simulink model "MAS_pc_up"  (R2022b)
settings: Solver=VariableStepAuto  StartTime=0.0  StopTime=300  RelTol=1e-3
values from neighbouring files (symbols this model uses):
  a1 = int8(3)    [init.m]
  A1 = [1.7,-1.3 ... (first row only)    [init.m]
  A2 = [1.8,-1.4 ... (first row only)    [init.m]
  a2 = int8(2)    [init.m]
  A3 = [1.4,-1.1 ... (first row only)    [init.m]
  a3 = int8(3)    [init.m]
  B1 = [1.0 ... (first row only)    [init.m]
  B2 = [1.7 ... (first row only)    [init.m]
  B3 = [0.8 ... (first row only)    [init.m]
  C1 = [1.0,0.3]    [init.m]
  C2 = [0.7,0.2]    [init.m]
  C3 = [1.1,0.4]    [init.m]
  F1 = [-0.4483 ... (first row only)    [init.m]
  F2 = [-0.6803 ... (first row only)    [init.m]
  F3 = [-0.3908 ... (first row only)    [init.m]
  G1 = -0.16    [init.m]
  G2 = -0.18    [init.m]
  G3 = -0.14    [init.m]
  H1 = -0.12    [init.m]
  H2 = -0.10    (= -0.1)    [init.m]
  H3 = -0.14    [init.m]
  M = [1,0,1 ... (first row only)    [init.m]
  s1 = int8(2)    [init.m]
  s2 = int8(3)    [init.m]
  s3 = int8(1)    [init.m]
  samp_t = 0.2    [init.m]
(part 1 of 2)
settings Model: Creator=Longct0  LastModifiedBy=Longct0

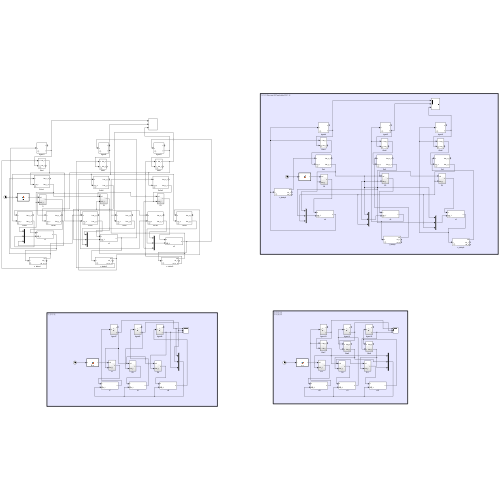
[thumbnail: Simulink's stored preview of the top-level diagram]
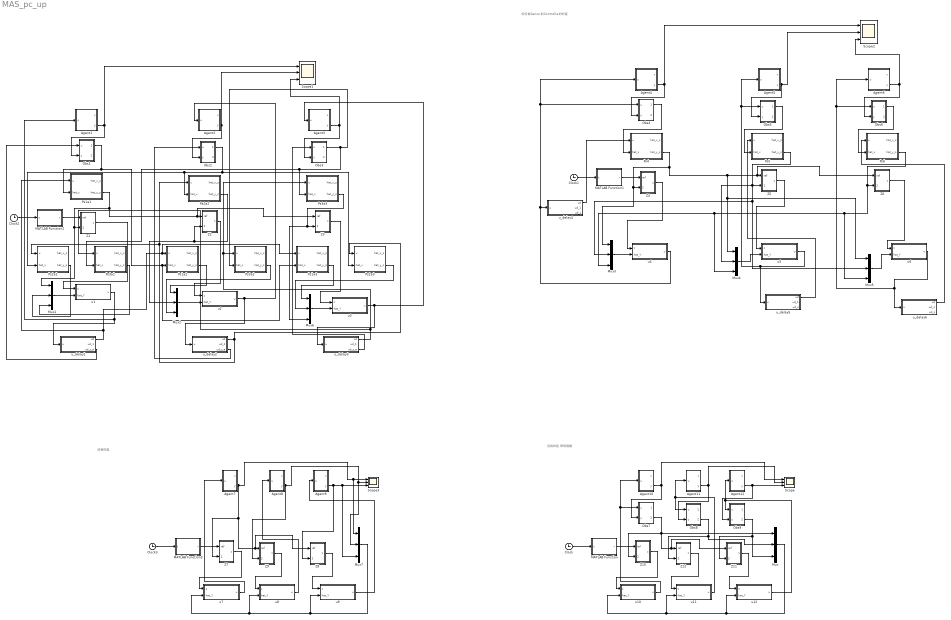
== system MAS_pc_up ==
  note: 仅仅有Sensor到Controller的时延
  note: 没有时延
      | 带观测器
  note: 没有时延
  Agent1 : Subsystem  mask{s=s1, a=a1}
      mask prompts: s "s-c"; a "c-a"
      mask DialogControl ParameterGroupVar Prompt: 参数
  Agent10 : Subsystem
  Agent11 : Subsystem
  Agent12 : Subsystem
  Agent2 : Subsystem  mask{s=s2, a=a2}
      mask prompts: s "s-c"; a "c-a"
      mask DialogControl ParameterGroupVar Prompt: 参数
  Agent3 : Subsystem  mask{s=s3, a=a3}
      mask prompts: s "s-c"; a "c-a"
      mask DialogControl ParameterGroupVar Prompt: 参数
  Agent4 : Subsystem  mask{s=s1, a=0}
      mask prompts: s "s-c"; a "c-a"
      mask DialogControl ParameterGroupVar Prompt: 参数
  Agent5 : Subsystem  mask{s=s2, a=0}
      mask prompts: s "s-c"; a "c-a"
      mask DialogControl ParameterGroupVar Prompt: 参数
  Agent6 : Subsystem  mask{s=s3, a=0}
      mask prompts: s "s-c"; a "c-a"
      mask DialogControl ParameterGroupVar Prompt: 参数
  Agent7 : Subsystem
  Agent8 : Subsystem
  Agent9 : Subsystem
  Clock{,1..3} (4 alike) : Clock
  MATLAB Function : MATLAB Function  TreatAsAtomicUnit=on
  MATLAB Function1 : MATLAB Function  TreatAsAtomicUnit=on
  MATLAB Function2 : MATLAB Function  TreatAsAtomicUnit=on
  MATLAB Function3 : MATLAB Function  TreatAsAtomicUnit=on
  Mux{,1..7} (8 alike) : Mux  Inputs=3
  Obs1 : Subsystem  mask{s=s1, a=a1}
      mask prompts: s "s-c"; a "c-a"
      mask DialogControl ParameterGroupVar Prompt: 参数
  Obs2 : Subsystem  mask{s=s2, a=a2}
      mask prompts: s "s-c"; a "c-a"
      mask DialogControl ParameterGroupVar Prompt: 参数
  Obs3 : Subsystem  mask{s=s3, a=a3}
      mask prompts: s "s-c"; a "c-a"
      mask DialogControl ParameterGroupVar Prompt: 参数
  Obs4 : Subsystem  mask{s=s1, a=a1}
      mask prompts: s "s-c"; a "c-a"
      mask DialogControl ParameterGroupVar Prompt: 参数
  Obs5 : Subsystem  mask{s=s2, a=a2}
      mask prompts: s "s-c"; a "c-a"
      mask DialogControl ParameterGroupVar Prompt: 参数
  Obs6 : Subsystem  mask{s=s3, a=a3}
      mask prompts: s "s-c"; a "c-a"
      mask DialogControl ParameterGroupVar Prompt: 参数
  Obs7 : Subsystem
  Obs8 : Subsystem
  Obs9 : Subsystem
  Ps1a1 : Subsystem  mask{s=s1, a=a1}
      mask prompts: s "s-c"; a "c-a"
      mask DialogControl ParameterGroupVar Prompt: 参数
  Ps1a2 : Subsystem  mask{s=s1, a=a2}
      mask prompts: s "s-c"; a "c-a"
      mask DialogControl ParameterGroupVar Prompt: 参数
  Ps1a3 : Subsystem  mask{s=s1, a=a3}
      mask prompts: s "s-c"; a "c-a"
      mask DialogControl ParameterGroupVar Prompt: 参数
  Ps2a1 : Subsystem  mask{s=s2, a=a1}
      mask prompts: s "s-c"; a "c-a"
      mask DialogControl ParameterGroupVar Prompt: 参数
  Ps2a2 : Subsystem  mask{s=s2, a=a2}
      mask prompts: s "s-c"; a "c-a"
      mask DialogControl ParameterGroupVar Prompt: 参数
  Ps2a3 : Subsystem  mask{s=s2, a=a3}
      mask prompts: s "s-c"; a "c-a"
      mask DialogControl ParameterGroupVar Prompt: 参数
  Ps3a1 : Subsystem  mask{s=s3, a=a1}
      mask prompts: s "s-c"; a "c-a"
      mask DialogControl ParameterGroupVar Prompt: 参数
  Ps3a2 : Subsystem  mask{s=s3, a=a2}
      mask prompts: s "s-c"; a "c-a"
      mask DialogControl ParameterGroupVar Prompt: 参数
  Ps3a3 : Subsystem  mask{s=s3, a=a3}
      mask prompts: s "s-c"; a "c-a"
      mask DialogControl ParameterGroupVar Prompt: 参数
  Ps4 : Subsystem  mask{s=s1, a=a1}
      mask prompts: s "s-c"; a "c-a"
      mask DialogControl ParameterGroupVar Prompt: 参数
  Ps5 : Subsystem  mask{s=s2, a=a2}
      mask prompts: s "s-c"; a "c-a"
      mask DialogControl ParameterGroupVar Prompt: 参数
  Ps6 : Subsystem  mask{s=s3, a=a3}
      mask prompts: s "s-c"; a "c-a"
      mask DialogControl ParameterGroupVar Prompt: 参数
  Scope{,1..3} (4 alike) : Scope  NumInputPorts=3
  Z1 : Subsystem
  Z10 : Subsystem
  Z11 : Subsystem
  Z12 : Subsystem
  Z2 : Subsystem
  Z3 : Subsystem
  Z4 : Subsystem
  Z5 : Subsystem
  Z6 : Subsystem
  Z7 : Subsystem
  Z8 : Subsystem
  Z9 : Subsystem
  u1 : Subsystem  mask{id=1}
      mask DialogControl ParameterGroupVar Prompt: 参数
  u10 : Subsystem  mask{id=1}
      mask DialogControl ParameterGroupVar Prompt: 参数
  u11 : Subsystem  mask{id=2}
      mask DialogControl ParameterGroupVar Prompt: 参数
  u12 : Subsystem  mask{id=3}
      mask DialogControl ParameterGroupVar Prompt: 参数
  u2 : Subsystem  mask{id=2}
      mask DialogControl ParameterGroupVar Prompt: 参数
  u3 : Subsystem  mask{id=3}
      mask DialogControl ParameterGroupVar Prompt: 参数
  u4 : Subsystem  mask{id=1}
      mask DialogControl ParameterGroupVar Prompt: 参数
  u5 : Subsystem  mask{id=2}
      mask DialogControl ParameterGroupVar Prompt: 参数
  u6 : Subsystem  mask{id=3}
      mask DialogControl ParameterGroupVar Prompt: 参数
  u7 : Subsystem  mask{id=1}
      mask DialogControl ParameterGroupVar Prompt: 参数
  u8 : Subsystem  mask{id=2}
      mask DialogControl ParameterGroupVar Prompt: 参数
  u9 : Subsystem  mask{id=3}
      mask DialogControl ParameterGroupVar Prompt: 参数
  u_delay1 : Subsystem  mask{s=s1, a=a1}
      mask prompts: s "s-c"; a "c-a"
      mask DialogControl ParameterGroupVar Prompt: 参数
  u_delay2 : Subsystem  mask{s=s2, a=a2}
      mask prompts: s "s-c"; a "c-a"
      mask DialogControl ParameterGroupVar Prompt: 参数
  u_delay3 : Subsystem  mask{s=s3, a=a3}
      mask prompts: s "s-c"; a "c-a"
      mask DialogControl ParameterGroupVar Prompt: 参数
  u_delay4 : Subsystem  mask{s=s1, a=a1}
      mask prompts: s "s-c"; a "c-a"
      mask DialogControl ParameterGroupVar Prompt: 参数
  u_delay5 : Subsystem  mask{s=s2, a=a2}
      mask prompts: s "s-c"; a "c-a"
      mask DialogControl ParameterGroupVar Prompt: 参数
  u_delay6 : Subsystem  mask{s=s3, a=a3}
      mask prompts: s "s-c"; a "c-a"
      mask DialogControl ParameterGroupVar Prompt: 参数
  wires:
  u6/1(u) -> Agent6/1(u), Obs6/1(u), u_delay6/1(u)
  u9/1(u) -> Agent9/1(u)
  Mux2/1 -> u2/2(hat_Y)
  Ps1a2/2(hat_y_s) -> Mux2/1
  MATLAB Function3/1(r) -> Z7/1(ref)
  Agent2/2(y) -> Obs2/2(y), Scope1/2
  Ps3a2/2(hat_y_s) -> Mux2/3
  Z9/1(z) -> u8/1(z)
  u2/1(u) -> Agent2/1(u), u_delay2/1(u)
  u3/1(u) -> Agent3/1(u), u_delay3/1(u)
  u_delay1/1(ud) -> Ps1a3/1(u), Ps1a2/1(u), Ps1a1/1(u)
  Mux1/1 -> u1/2(hat_Y)
  Obs5/1(hat_x) -> Ps5/2(hat_x)
  Obs3/1(hat_x) -> Ps3a3/2(hat_x), Ps3a1/2(hat_x), Ps3a2/2(hat_x)
  Ps3a3/2(hat_y_s) -> Mux6/3, Z3/2(hat_y)
  Agent1/2(y) -> Scope1/1, Obs1/2(y)
  MATLAB Function2/1(r) -> Z1/1(ref)
  Ps3a1/2(hat_y_s) -> Mux1/3
  Ps1a1/2(hat_y_s) -> Z3/1(ref), Z2/1(ref), Mux1/1, Z1/2(hat_y)
  u1/1(u) -> Agent1/1(u), u_delay1/1(u)
  Ps5/2(hat_y_s) -> Mux5/2, Mux3/2, Z5/2(hat_y), Mux4/2
  Mux3/1 -> u4/2(hat_Y)
  Clock2/1 -> MATLAB Function2/1(t)
  Mux5/1 -> u6/2(hat_Y)
  Obs1/1(hat_x) -> Ps1a3/2(hat_x), Ps1a2/2(hat_x), Ps1a1/2(hat_x)
  u5/1(u) -> Agent5/1(u), Obs5/1(u), u_delay5/1(u)
  Agent4/2(y) -> Scope2/1, Obs4/2(y)
  Clock1/1 -> MATLAB Function1/1(t)
  Ps4/2(hat_y_s) -> Mux4/1, Mux5/1, Z6/1(ref), Z5/1(ref), Mux3/1, Z4/2(hat_y)
  Obs6/1(hat_x) -> Ps6/2(hat_x)
  u4/1(u) -> u_delay4/1(u), Obs4/1(u), Agent4/1(u)
  Z4/1(z) -> u4/1(z)
  Agent6/2(y) -> Obs6/2(y), Scope2/3
  MATLAB Function1/1(r) -> Z4/1(ref)
  Agent3/2(y) -> Obs3/2(y), Scope1/3
  Ps2a3/2(hat_y_s) -> Mux6/2
  Ps2a1/2(hat_y_s) -> Mux1/2
  u_delay6/1(ud) -> Ps6/1(u)
  Agent7/2(y) -> Z8/1(ref), Z9/1(ref), Z7/2(hat_y), Mux7/1, Scope3/1
  u_delay2/1(ud) -> Ps2a3/1(u), Ps2a2/1(u), Ps2a1/1(u)
  Z1/1(z) -> u1/1(z)
  Z7/1(z) -> u7/1(z)
  Mux/1 -> u12/2(hat_Y), u10/2(hat_Y), u11/2(hat_Y)
  Mux7/1 -> u9/2(hat_Y), u7/2(hat_Y), u8/2(hat_Y)
  u_delay4/1(ud) -> Ps4/1(u)
  Z6/1(z) -> u6/1(z)
  Ps2a2/2(hat_y_s) -> Mux2/2, Z2/2(hat_y)
  u_delay1/3(ud_s_a) -> Obs1/1(u)
  Ps6/2(hat_y_s) -> Mux4/3, Mux3/3, Mux5/3, Z6/2(hat_y)
  Clock3/1 -> MATLAB Function3/1(t)
  u7/1(u) -> Agent7/1(u)
  u_delay2/3(ud_s_a) -> Obs2/1(u)
  Z2/1(z) -> u2/1(z)
  MATLAB Function/1(r) -> Z10/1(ref)
  Z12/1(z) -> u11/1(z)
  Obs9/2(hat_y) -> Mux/3, Z11/2(hat_y)
  u10/1(u) -> Agent10/1(u), Obs7/1(u)
  Agent8/2(y) -> Z9/2(hat_y), Mux7/2, Scope3/2
  u_delay3/1(ud) -> Ps3a1/1(u), Ps3a3/1(u), Ps3a2/1(u)
  Ps1a3/2(hat_y_s) -> Mux6/1
  Clock/1 -> MATLAB Function/1(t)
  Mux4/1 -> u5/2(hat_Y)
  Agent12/2(y) -> Scope/3, Obs9/2(y)
  Obs8/2(hat_y) -> Mux/2, Z12/2(hat_y)
  Z11/1(z) -> u12/1(z)
  Agent5/2(y) -> Obs5/2(y), Scope2/2
  Z3/1(z) -> u3/1(z)
  Z5/1(z) -> u5/1(z)
  Obs2/1(hat_x) -> Ps2a1/2(hat_x), Ps2a2/2(hat_x), Ps2a3/2(hat_x)
  Obs4/1(hat_x) -> Ps4/2(hat_x)
  Agent10/2(y) -> Scope/1, Obs7/2(y)
  Mux6/1 -> u3/2(hat_Y)
  Agent9/2(y) -> Z8/2(hat_y), Scope3/3, Mux7/3
  u_delay3/3(ud_s_a) -> Obs3/1(u)
  Obs7/2(hat_y) -> Mux/1, Z11/1(ref), Z12/1(ref), Z10/2(hat_y)
  u11/1(u) -> Agent11/1(u), Obs8/1(u)
  Z8/1(z) -> u9/1(z)
  u12/1(u) -> Agent12/1(u), Obs9/1(u)
  Agent11/2(y) -> Scope/2, Obs8/2(y)
  u_delay5/1(ud) -> Ps5/1(u)
  Z10/1(z) -> u10/1(z)
  u8/1(u) -> Agent8/1(u)

== system MAS_pc_up/Agent1 ==
  u : Inport
  A : Constant  Value=A1  VectorParams1D=off
  Add : Sum
  B : Constant  Value=B1  VectorParams1D=off
  C : Constant  Value=C1  VectorParams1D=off
  Product : Product  Multiplication=Matrix(*)
  Product1 : Product  Multiplication=Matrix(*)
  Product2 : Product  Multiplication=Matrix(*)
  Unit Delay : UnitDelay  SampleTime=samp_t  HasFrameUpgradeWarning=on
  Variable Integer Delay : Delay  DelayLengthSource=Input port  SampleTime=samp_t
      settings: InputPortMap=u0,p1
  a : Constant  Value=a
  x : Outport
  y : Outport  Port=2
  wires:
  B/1 -> Product1/1
  Unit Delay/1 -> x/1, Product2/2, Product/2
  Product/1 -> Add/1
  Product1/1 -> Add/2
  A/1 -> Product/1
  Product2/1 -> y/1
  C/1 -> Product2/1
  Add/1 -> Unit Delay/1
  u/1 -> Variable Integer Delay/1
  Variable Integer Delay/1 -> Product1/2
  a/1 -> Variable Integer Delay/2

== system MAS_pc_up/Agent10 ==
  u : Inport
  A : Constant  Value=A1  VectorParams1D=off
  Add : Sum
  B : Constant  Value=B1  VectorParams1D=off
  C : Constant  Value=C1  VectorParams1D=off
  Product : Product  Multiplication=Matrix(*)
  Product1 : Product  Multiplication=Matrix(*)
  Product2 : Product  Multiplication=Matrix(*)
  Unit Delay : UnitDelay  SampleTime=-1  HasFrameUpgradeWarning=on
  x : Outport
  y : Outport  Port=2
  wires:
  B/1 -> Product1/1
  Unit Delay/1 -> x/1, Product2/2, Product/2
  Product/1 -> Add/1
  Product1/1 -> Add/2
  u/1 -> Product1/2
  A/1 -> Product/1
  Product2/1 -> y/1
  C/1 -> Product2/1
  Add/1 -> Unit Delay/1

== system MAS_pc_up/Agent11 ==
  u : Inport
  A : Constant  Value=A2  VectorParams1D=off
  Add : Sum
  B : Constant  Value=B2  VectorParams1D=off
  C : Constant  Value=C2  VectorParams1D=off
  Product : Product  Multiplication=Matrix(*)
  Product1 : Product  Multiplication=Matrix(*)
  Product2 : Product  Multiplication=Matrix(*)
  Unit Delay : UnitDelay  SampleTime=-1  HasFrameUpgradeWarning=on
  x : Outport
  y : Outport  Port=2
  wires:
  B/1 -> Product1/1
  Add/1 -> Unit Delay/1
  Unit Delay/1 -> x/1, Product2/2, Product/2
  Product/1 -> Add/1
  Product1/1 -> Add/2
  u/1 -> Product1/2
  A/1 -> Product/1
  Product2/1 -> y/1
  C/1 -> Product2/1

== system MAS_pc_up/Agent12 ==
  u : Inport
  A : Constant  Value=A3  VectorParams1D=off
  Add : Sum
  B : Constant  Value=B3  VectorParams1D=off
  C : Constant  Value=C3  VectorParams1D=off
  Product : Product  Multiplication=Matrix(*)
  Product1 : Product  Multiplication=Matrix(*)
  Product2 : Product  Multiplication=Matrix(*)
  Unit Delay : UnitDelay  SampleTime=-1  HasFrameUpgradeWarning=on
  x : Outport
  y : Outport  Port=2
  wires:
  B/1 -> Product1/1
  Add/1 -> Unit Delay/1
  Unit Delay/1 -> x/1, Product2/2, Product/2
  Product/1 -> Add/1
  Product1/1 -> Add/2
  u/1 -> Product1/2
  A/1 -> Product/1
  Product2/1 -> y/1
  C/1 -> Product2/1

== system MAS_pc_up/Agent2 ==
  u : Inport
  A : Constant  Value=A2  VectorParams1D=off
  Add : Sum
  B : Constant  Value=B2  VectorParams1D=off
  C : Constant  Value=C2  VectorParams1D=off
  Product : Product  Multiplication=Matrix(*)
  Product1 : Product  Multiplication=Matrix(*)
  Product2 : Product  Multiplication=Matrix(*)
  Unit Delay : UnitDelay  SampleTime=samp_t  HasFrameUpgradeWarning=on
  Variable Integer Delay : Delay  DelayLengthSource=Input port  SampleTime=samp_t
      settings: InputPortMap=u0,p1
  a : Constant  Value=a
  x : Outport
  y : Outport  Port=2
  wires:
  B/1 -> Product1/1
  Add/1 -> Unit Delay/1
  Unit Delay/1 -> x/1, Product2/2, Product/2
  Product/1 -> Add/1
  Product1/1 -> Add/2
  A/1 -> Product/1
  Product2/1 -> y/1
  C/1 -> Product2/1
  u/1 -> Variable Integer Delay/1
  Variable Integer Delay/1 -> Product1/2
  a/1 -> Variable Integer Delay/2

== system MAS_pc_up/Agent3 ==
  u : Inport
  A : Constant  Value=A3  VectorParams1D=off
  Add : Sum
  B : Constant  Value=B3  VectorParams1D=off
  C : Constant  Value=C3  VectorParams1D=off
  Product : Product  Multiplication=Matrix(*)
  Product1 : Product  Multiplication=Matrix(*)
  Product2 : Product  Multiplication=Matrix(*)
  Unit Delay : UnitDelay  SampleTime=samp_t  HasFrameUpgradeWarning=on
  Variable Integer Delay : Delay  DelayLengthSource=Input port  SampleTime=samp_t
      settings: InputPortMap=u0,p1
  a : Constant  Value=a
  x : Outport
  y : Outport  Port=2
  wires:
  B/1 -> Product1/1
  Add/1 -> Unit Delay/1
  Unit Delay/1 -> x/1, Product2/2, Product/2
  Product/1 -> Add/1
  Product1/1 -> Add/2
  A/1 -> Product/1
  Product2/1 -> y/1
  C/1 -> Product2/1
  u/1 -> Variable Integer Delay/1
  a/1 -> Variable Integer Delay/2
  Variable Integer Delay/1 -> Product1/2

== system MAS_pc_up/Agent4 ==
  u : Inport
  A : Constant  Value=A1  VectorParams1D=off
  Add : Sum
  B : Constant  Value=B1  VectorParams1D=off
  C : Constant  Value=C1  VectorParams1D=off
  Product : Product  Multiplication=Matrix(*)
  Product1 : Product  Multiplication=Matrix(*)
  Product2 : Product  Multiplication=Matrix(*)
  Unit Delay : UnitDelay  SampleTime=samp_t  HasFrameUpgradeWarning=on
  Variable Integer Delay : Delay  DelayLengthSource=Input port  SampleTime=samp_t
      settings: InputPortMap=u0,p1
  a : Constant  Value=a
  x : Outport
  y : Outport  Port=2
  wires:
  B/1 -> Product1/1
  Unit Delay/1 -> x/1, Product2/2, Product/2
  Product/1 -> Add/1
  Product1/1 -> Add/2
  A/1 -> Product/1
  Product2/1 -> y/1
  C/1 -> Product2/1
  Add/1 -> Unit Delay/1
  u/1 -> Variable Integer Delay/1
  Variable Integer Delay/1 -> Product1/2
  a/1 -> Variable Integer Delay/2

== system MAS_pc_up/Agent5 ==
  u : Inport
  A : Constant  Value=A2  VectorParams1D=off
  Add : Sum
  B : Constant  Value=B2  VectorParams1D=off
  C : Constant  Value=C2  VectorParams1D=off
  Product : Product  Multiplication=Matrix(*)
  Product1 : Product  Multiplication=Matrix(*)
  Product2 : Product  Multiplication=Matrix(*)
  Unit Delay : UnitDelay  SampleTime=samp_t  HasFrameUpgradeWarning=on
  Variable Integer Delay : Delay  DelayLengthSource=Input port  SampleTime=samp_t
      settings: InputPortMap=u0,p1
  a : Constant  Value=a
  x : Outport
  y : Outport  Port=2
  wires:
  B/1 -> Product1/1
  Add/1 -> Unit Delay/1
  Unit Delay/1 -> x/1, Product2/2, Product/2
  Product/1 -> Add/1
  Product1/1 -> Add/2
  A/1 -> Product/1
  Product2/1 -> y/1
  C/1 -> Product2/1
  u/1 -> Variable Integer Delay/1
  Variable Integer Delay/1 -> Product1/2
  a/1 -> Variable Integer Delay/2

== system MAS_pc_up/Agent6 ==
  u : Inport
  A : Constant  Value=A3  VectorParams1D=off
  Add : Sum
  B : Constant  Value=B3  VectorParams1D=off
  C : Constant  Value=C3  VectorParams1D=off
  Product : Product  Multiplication=Matrix(*)
  Product1 : Product  Multiplication=Matrix(*)
  Product2 : Product  Multiplication=Matrix(*)
  Unit Delay : UnitDelay  SampleTime=samp_t  HasFrameUpgradeWarning=on
  Variable Integer Delay : Delay  DelayLengthSource=Input port  SampleTime=samp_t
      settings: InputPortMap=u0,p1
  a : Constant  Value=a
  x : Outport
  y : Outport  Port=2
  wires:
  B/1 -> Product1/1
  Add/1 -> Unit Delay/1
  Unit Delay/1 -> x/1, Product2/2, Product/2
  Product/1 -> Add/1
  Product1/1 -> Add/2
  A/1 -> Product/1
  Product2/1 -> y/1
  C/1 -> Product2/1
  u/1 -> Variable Integer Delay/1
  a/1 -> Variable Integer Delay/2
  Variable Integer Delay/1 -> Product1/2

== system MAS_pc_up/Agent7 ==
  u : Inport
  A : Constant  Value=A1  VectorParams1D=off
  Add : Sum
  B : Constant  Value=B1  VectorParams1D=off
  C : Constant  Value=C1  VectorParams1D=off
  Product : Product  Multiplication=Matrix(*)
  Product1 : Product  Multiplication=Matrix(*)
  Product2 : Product  Multiplication=Matrix(*)
  Unit Delay : UnitDelay  SampleTime=samp_t  HasFrameUpgradeWarning=on
  x : Outport
  y : Outport  Port=2
  wires:
  B/1 -> Product1/1
  Unit Delay/1 -> x/1, Product2/2, Product/2
  Product/1 -> Add/1
  Product1/1 -> Add/2
  u/1 -> Product1/2
  A/1 -> Product/1
  Product2/1 -> y/1
  C/1 -> Product2/1
  Add/1 -> Unit Delay/1

== system MAS_pc_up/Agent8 ==
  u : Inport
  A : Constant  Value=A2  VectorParams1D=off
  Add : Sum
  B : Constant  Value=B2  VectorParams1D=off
  C : Constant  Value=C2  VectorParams1D=off
  Product : Product  Multiplication=Matrix(*)
  Product1 : Product  Multiplication=Matrix(*)
  Product2 : Product  Multiplication=Matrix(*)
  Unit Delay : UnitDelay  SampleTime=samp_t  HasFrameUpgradeWarning=on
  x : Outport
  y : Outport  Port=2
  wires:
  B/1 -> Product1/1
  Add/1 -> Unit Delay/1
  Unit Delay/1 -> x/1, Product2/2, Product/2
  Product/1 -> Add/1
  Product1/1 -> Add/2
  u/1 -> Product1/2
  A/1 -> Product/1
  Product2/1 -> y/1
  C/1 -> Product2/1

== system MAS_pc_up/Agent9 ==
  u : Inport
  A : Constant  Value=A3  VectorParams1D=off
  Add : Sum
  B : Constant  Value=B3  VectorParams1D=off
  C : Constant  Value=C3  VectorParams1D=off
  Product : Product  Multiplication=Matrix(*)
  Product1 : Product  Multiplication=Matrix(*)
  Product2 : Product  Multiplication=Matrix(*)
  Unit Delay : UnitDelay  SampleTime=samp_t  HasFrameUpgradeWarning=on
  x : Outport
  y : Outport  Port=2
  wires:
  B/1 -> Product1/1
  Add/1 -> Unit Delay/1
  Unit Delay/1 -> x/1, Product2/2, Product/2
  Product/1 -> Add/1
  Product1/1 -> Add/2
  u/1 -> Product1/2
  A/1 -> Product/1
  Product2/1 -> y/1
  C/1 -> Product2/1

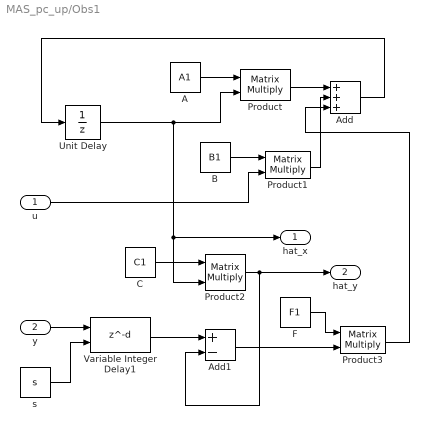
== system MAS_pc_up/Obs1 ==
  u : Inport
  y : Inport  Port=2
  A : Constant  Value=A1  VectorParams1D=off
  Add : Sum  Inputs=+++
  Add1 : Sum  Inputs=+-
  B : Constant  Value=B1  VectorParams1D=off
  C : Constant  Value=C1  VectorParams1D=off
  F : Constant  Value=F1  VectorParams1D=off
  Product{,1..3} (4 alike) : Product  Multiplication=Matrix(*)
  Unit Delay : UnitDelay  SampleTime=samp_t  HasFrameUpgradeWarning=on
  Variable Integer Delay1 : Delay  DelayLengthSource=Input port  SampleTime=samp_t
      settings: InputPortMap=u0,p1
  s : Constant  Value=s
  hat_x : Outport
  hat_y : Outport  Port=2
  wires:
  B/1 -> Product1/1
  Add/1 -> Unit Delay/1
  Unit Delay/1 -> Product/2, hat_x/1, Product2/2
  Product/1 -> Add/1
  Product1/1 -> Add/2
  A/1 -> Product/1
  Product2/1 -> Add1/2, hat_y/1
  Add1/1 -> Product3/2
  F/1 -> Product3/1
  Product3/1 -> Add/3
  C/1 -> Product2/1
  y/1 -> Variable Integer Delay1/1
  Variable Integer Delay1/1 -> Add1/1
  s/1 -> Variable Integer Delay1/2
  u/1 -> Product1/2

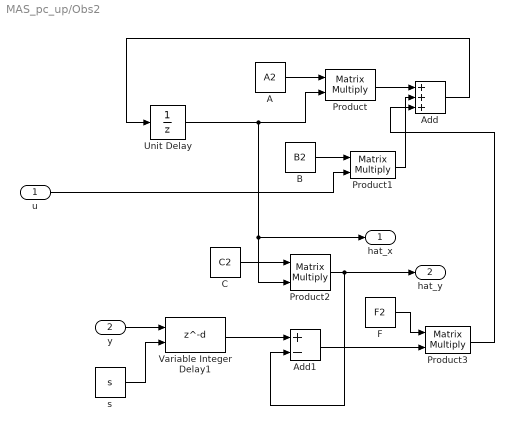
== system MAS_pc_up/Obs2 ==
  u : Inport
  y : Inport  Port=2
  A : Constant  Value=A2  VectorParams1D=off
  Add : Sum  Inputs=+++
  Add1 : Sum  Inputs=+-
  B : Constant  Value=B2  VectorParams1D=off
  C : Constant  Value=C2  VectorParams1D=off
  F : Constant  Value=F2  VectorParams1D=off
  Product{,1..3} (4 alike) : Product  Multiplication=Matrix(*)
  Unit Delay : UnitDelay  SampleTime=samp_t  HasFrameUpgradeWarning=on
  Variable Integer Delay1 : Delay  DelayLengthSource=Input port  SampleTime=samp_t
      settings: InputPortMap=u0,p1
  s : Constant  Value=s
  hat_x : Outport
  hat_y : Outport  Port=2
  wires:
  B/1 -> Product1/1
  Add/1 -> Unit Delay/1
  Unit Delay/1 -> Product/2, Product2/2, hat_x/1
  Product/1 -> Add/1
  Product1/1 -> Add/2
  A/1 -> Product/1
  Product2/1 -> Add1/2, hat_y/1
  Add1/1 -> Product3/2
  F/1 -> Product3/1
  Product3/1 -> Add/3
  C/1 -> Product2/1
  s/1 -> Variable Integer Delay1/2
  y/1 -> Variable Integer Delay1/1
  Variable Integer Delay1/1 -> Add1/1
  u/1 -> Product1/2

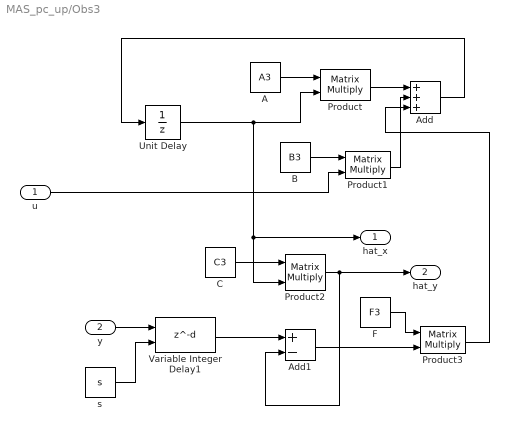
== system MAS_pc_up/Obs3 ==
  u : Inport
  y : Inport  Port=2
  A : Constant  Value=A3  VectorParams1D=off
  Add : Sum  Inputs=+++
  Add1 : Sum  Inputs=+-
  B : Constant  Value=B3  VectorParams1D=off
  C : Constant  Value=C3  VectorParams1D=off
  F : Constant  Value=F3  VectorParams1D=off
  Product{,1..3} (4 alike) : Product  Multiplication=Matrix(*)
  Unit Delay : UnitDelay  SampleTime=samp_t  HasFrameUpgradeWarning=on
  Variable Integer Delay1 : Delay  DelayLengthSource=Input port  SampleTime=samp_t
      settings: InputPortMap=u0,p1
  s : Constant  Value=s
  hat_x : Outport
  hat_y : Outport  Port=2
  wires:
  B/1 -> Product1/1
  Add/1 -> Unit Delay/1
  Unit Delay/1 -> Product/2, hat_x/1, Product2/2
  Product/1 -> Add/1
  Product1/1 -> Add/2
  A/1 -> Product/1
  Product2/1 -> Add1/2, hat_y/1
  Add1/1 -> Product3/2
  F/1 -> Product3/1
  Product3/1 -> Add/3
  C/1 -> Product2/1
  s/1 -> Variable Integer Delay1/2
  y/1 -> Variable Integer Delay1/1
  Variable Integer Delay1/1 -> Add1/1
  u/1 -> Product1/2

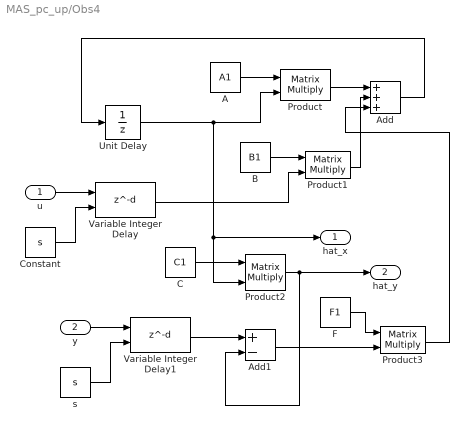
== system MAS_pc_up/Obs4 ==
  u : Inport
  y : Inport  Port=2
  A : Constant  Value=A1  VectorParams1D=off
  Add : Sum  Inputs=+++
  Add1 : Sum  Inputs=+-
  B : Constant  Value=B1  VectorParams1D=off
  C : Constant  Value=C1  VectorParams1D=off
  Constant : Constant  Value=s
  F : Constant  Value=F1  VectorParams1D=off
  Product{,1..3} (4 alike) : Product  Multiplication=Matrix(*)
  Unit Delay : UnitDelay  SampleTime=samp_t  HasFrameUpgradeWarning=on
  Variable Integer Delay : Delay  DelayLengthSource=Input port  SampleTime=samp_t
      settings: InputPortMap=u0,p1
  Variable Integer Delay1 : Delay  DelayLengthSource=Input port  SampleTime=samp_t
      settings: InputPortMap=u0,p1
  s : Constant  Value=s
  hat_x : Outport
  hat_y : Outport  Port=2
  wires:
  B/1 -> Product1/1
  Add/1 -> Unit Delay/1
  Unit Delay/1 -> Product/2, hat_x/1, Product2/2
  Product/1 -> Add/1
  Product1/1 -> Add/2
  A/1 -> Product/1
  Product2/1 -> Add1/2, hat_y/1
  Add1/1 -> Product3/2
  F/1 -> Product3/1
  Product3/1 -> Add/3
  C/1 -> Product2/1
  u/1 -> Variable Integer Delay/1
  Variable Integer Delay/1 -> Product1/2
  Constant/1 -> Variable Integer Delay/2
  y/1 -> Variable Integer Delay1/1
  Variable Integer Delay1/1 -> Add1/1
  s/1 -> Variable Integer Delay1/2

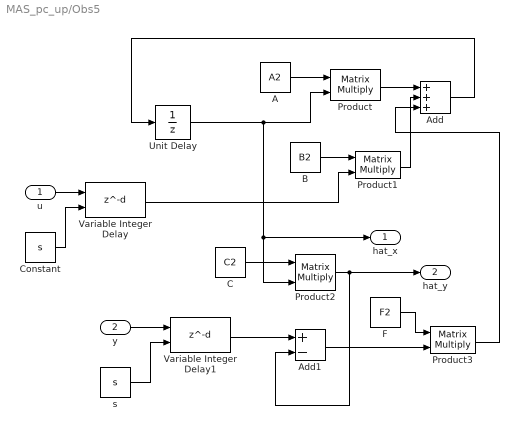
== system MAS_pc_up/Obs5 ==
  u : Inport
  y : Inport  Port=2
  A : Constant  Value=A2  VectorParams1D=off
  Add : Sum  Inputs=+++
  Add1 : Sum  Inputs=+-
  B : Constant  Value=B2  VectorParams1D=off
  C : Constant  Value=C2  VectorParams1D=off
  Constant : Constant  Value=s
  F : Constant  Value=F2  VectorParams1D=off
  Product{,1..3} (4 alike) : Product  Multiplication=Matrix(*)
  Unit Delay : UnitDelay  SampleTime=samp_t  HasFrameUpgradeWarning=on
  Variable Integer Delay : Delay  DelayLengthSource=Input port  SampleTime=samp_t
      settings: InputPortMap=u0,p1
  Variable Integer Delay1 : Delay  DelayLengthSource=Input port  SampleTime=samp_t
      settings: InputPortMap=u0,p1
  s : Constant  Value=s
  hat_x : Outport
  hat_y : Outport  Port=2
  wires:
  B/1 -> Product1/1
  Add/1 -> Unit Delay/1
  Unit Delay/1 -> Product/2, Product2/2, hat_x/1
  Product/1 -> Add/1
  Product1/1 -> Add/2
  A/1 -> Product/1
  Product2/1 -> Add1/2, hat_y/1
  Add1/1 -> Product3/2
  F/1 -> Product3/1
  Product3/1 -> Add/3
  C/1 -> Product2/1
  Constant/1 -> Variable Integer Delay/2
  u/1 -> Variable Integer Delay/1
  Variable Integer Delay/1 -> Product1/2
  s/1 -> Variable Integer Delay1/2
  y/1 -> Variable Integer Delay1/1
  Variable Integer Delay1/1 -> Add1/1

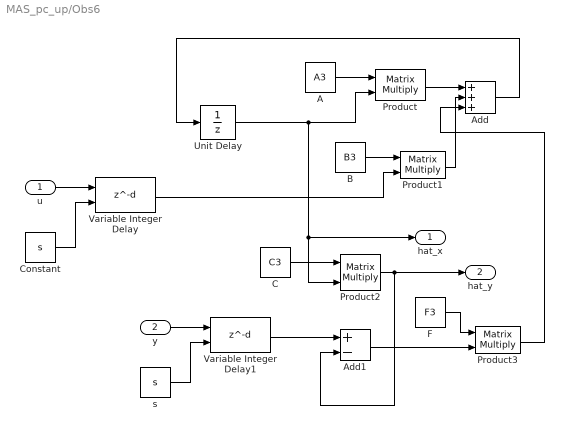
== system MAS_pc_up/Obs6 ==
  u : Inport
  y : Inport  Port=2
  A : Constant  Value=A3  VectorParams1D=off
  Add : Sum  Inputs=+++
  Add1 : Sum  Inputs=+-
  B : Constant  Value=B3  VectorParams1D=off
  C : Constant  Value=C3  VectorParams1D=off
  Constant : Constant  Value=s
  F : Constant  Value=F3  VectorParams1D=off
  Product{,1..3} (4 alike) : Product  Multiplication=Matrix(*)
  Unit Delay : UnitDelay  SampleTime=samp_t  HasFrameUpgradeWarning=on
  Variable Integer Delay : Delay  DelayLengthSource=Input port  SampleTime=samp_t
      settings: InputPortMap=u0,p1
  Variable Integer Delay1 : Delay  DelayLengthSource=Input port  SampleTime=samp_t
      settings: InputPortMap=u0,p1
  s : Constant  Value=s
  hat_x : Outport
  hat_y : Outport  Port=2
  wires:
  B/1 -> Product1/1
  Add/1 -> Unit Delay/1
  Unit Delay/1 -> Product/2, hat_x/1, Product2/2
  Product/1 -> Add/1
  Product1/1 -> Add/2
  A/1 -> Product/1
  Product2/1 -> Add1/2, hat_y/1
  Add1/1 -> Product3/2
  F/1 -> Product3/1
  Product3/1 -> Add/3
  C/1 -> Product2/1
  Constant/1 -> Variable Integer Delay/2
  u/1 -> Variable Integer Delay/1
  Variable Integer Delay/1 -> Product1/2
  s/1 -> Variable Integer Delay1/2
  y/1 -> Variable Integer Delay1/1
  Variable Integer Delay1/1 -> Add1/1

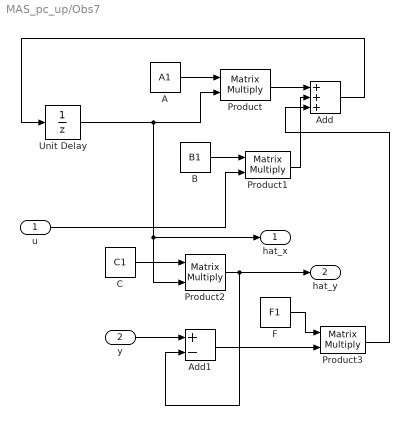
== system MAS_pc_up/Obs7 ==
  u : Inport
  y : Inport  Port=2
  A : Constant  Value=A1  VectorParams1D=off
  Add : Sum  Inputs=+++
  Add1 : Sum  Inputs=+-
  B : Constant  Value=B1  VectorParams1D=off
  C : Constant  Value=C1  VectorParams1D=off
  F : Constant  Value=F1  VectorParams1D=off
  Product{,1..3} (4 alike) : Product  Multiplication=Matrix(*)
  Unit Delay : UnitDelay  SampleTime=-1  HasFrameUpgradeWarning=on
  hat_x : Outport
  hat_y : Outport  Port=2
  wires:
  B/1 -> Product1/1
  Add/1 -> Unit Delay/1
  Unit Delay/1 -> Product/2, hat_x/1, Product2/2
  Product/1 -> Add/1
  Product1/1 -> Add/2
  u/1 -> Product1/2
  A/1 -> Product/1
  Product2/1 -> Add1/2, hat_y/1
  y/1 -> Add1/1
  Add1/1 -> Product3/2
  F/1 -> Product3/1
  Product3/1 -> Add/3
  C/1 -> Product2/1

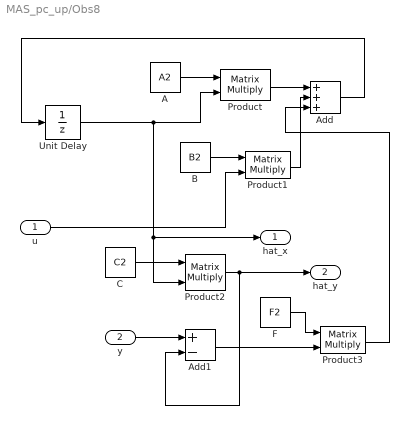
== system MAS_pc_up/Obs8 ==
  u : Inport
  y : Inport  Port=2
  A : Constant  Value=A2  VectorParams1D=off
  Add : Sum  Inputs=+++
  Add1 : Sum  Inputs=+-
  B : Constant  Value=B2  VectorParams1D=off
  C : Constant  Value=C2  VectorParams1D=off
  F : Constant  Value=F2  VectorParams1D=off
  Product{,1..3} (4 alike) : Product  Multiplication=Matrix(*)
  Unit Delay : UnitDelay  SampleTime=-1  HasFrameUpgradeWarning=on
  hat_x : Outport
  hat_y : Outport  Port=2
  wires:
  B/1 -> Product1/1
  Add/1 -> Unit Delay/1
  Unit Delay/1 -> Product/2, Product2/2, hat_x/1
  Product/1 -> Add/1
  Product1/1 -> Add/2
  u/1 -> Product1/2
  A/1 -> Product/1
  Product2/1 -> Add1/2, hat_y/1
  y/1 -> Add1/1
  Add1/1 -> Product3/2
  F/1 -> Product3/1
  Product3/1 -> Add/3
  C/1 -> Product2/1

== system MAS_pc_up/Obs9 ==
  u : Inport
  y : Inport  Port=2
  A : Constant  Value=A3  VectorParams1D=off
  Add : Sum  Inputs=+++
  Add1 : Sum  Inputs=+-
  B : Constant  Value=B3  VectorParams1D=off
  C : Constant  Value=C3  VectorParams1D=off
  F : Constant  Value=F3  VectorParams1D=off
  Product{,1..3} (4 alike) : Product  Multiplication=Matrix(*)
  Unit Delay : UnitDelay  SampleTime=-1  HasFrameUpgradeWarning=on
  hat_x : Outport
  hat_y : Outport  Port=2
  wires:
  B/1 -> Product1/1
  Add/1 -> Unit Delay/1
  Unit Delay/1 -> Product/2, hat_x/1, Product2/2
  Product/1 -> Add/1
  Product1/1 -> Add/2
  u/1 -> Product1/2
  A/1 -> Product/1
  Product2/1 -> Add1/2, hat_y/1
  y/1 -> Add1/1
  Add1/1 -> Product3/2
  F/1 -> Product3/1
  Product3/1 -> Add/3
  C/1 -> Product2/1

== system MAS_pc_up/Ps1a1 ==
  u : Inport
  hat_x : Inport  Port=2
  A : Constant  Value=A1  VectorParams1D=off
  B : Constant  Value=B1  VectorParams1D=off
  C : Constant  Value=C1  VectorParams1D=off
  Demux : Demux  Outputs=10
  MATLAB Function : MATLAB Function  TreatAsAtomicUnit=on
  a : Constant  Value=a
  s : Constant  Value=s
  hat_x_s : Outport
  hat_y_s : Outport  Port=2
  wires:
  MATLAB Function/2(y) -> hat_y_s/1
  MATLAB Function/1(x_) -> hat_x_s/1
  hat_x/1 -> MATLAB Function/11(x)
  A/1 -> MATLAB Function/14(A)
  B/1 -> MATLAB Function/15(B)
  C/1 -> MATLAB Function/16(C)
  u/1 -> Demux/1
  s/1 -> MATLAB Function/12(s)
  a/1 -> MATLAB Function/13(a)
  Demux/1 -> MATLAB Function/1(u10)
  Demux/2 -> MATLAB Function/2(u9)
  Demux/3 -> MATLAB Function/3(u8)
  Demux/4 -> MATLAB Function/4(u7)
  Demux/5 -> MATLAB Function/5(u6)
  Demux/6 -> MATLAB Function/6(u5)
  Demux/7 -> MATLAB Function/7(u4)
  Demux/8 -> MATLAB Function/8(u3)
  Demux/9 -> MATLAB Function/9(u2)
  Demux/10 -> MATLAB Function/10(u1)

== system MAS_pc_up/Ps1a2 ==
  u : Inport
  hat_x : Inport  Port=2
  A : Constant  Value=A1  VectorParams1D=off
  B : Constant  Value=B1  VectorParams1D=off
  C : Constant  Value=C1  VectorParams1D=off
  Demux : Demux  Outputs=10
  MATLAB Function : MATLAB Function  TreatAsAtomicUnit=on
  a : Constant  Value=a
  s : Constant  Value=s
  hat_x_s : Outport
  hat_y_s : Outport  Port=2
  wires:
  MATLAB Function/2(y) -> hat_y_s/1
  MATLAB Function/1(x_) -> hat_x_s/1
  hat_x/1 -> MATLAB Function/11(x)
  A/1 -> MATLAB Function/14(A)
  B/1 -> MATLAB Function/15(B)
  C/1 -> MATLAB Function/16(C)
  u/1 -> Demux/1
  s/1 -> MATLAB Function/12(s)
  a/1 -> MATLAB Function/13(a)
  Demux/1 -> MATLAB Function/1(u10)
  Demux/2 -> MATLAB Function/2(u9)
  Demux/3 -> MATLAB Function/3(u8)
  Demux/4 -> MATLAB Function/4(u7)
  Demux/5 -> MATLAB Function/5(u6)
  Demux/6 -> MATLAB Function/6(u5)
  Demux/7 -> MATLAB Function/7(u4)
  Demux/8 -> MATLAB Function/8(u3)
  Demux/9 -> MATLAB Function/9(u2)
  Demux/10 -> MATLAB Function/10(u1)

== system MAS_pc_up/Ps1a3 ==
  u : Inport
  hat_x : Inport  Port=2
  A : Constant  Value=A1  VectorParams1D=off
  B : Constant  Value=B1  VectorParams1D=off
  C : Constant  Value=C1  VectorParams1D=off
  Demux : Demux  Outputs=10
  MATLAB Function : MATLAB Function  TreatAsAtomicUnit=on
  a : Constant  Value=a
  s : Constant  Value=s
  hat_x_s : Outport
  hat_y_s : Outport  Port=2
  wires:
  MATLAB Function/2(y) -> hat_y_s/1
  MATLAB Function/1(x_) -> hat_x_s/1
  hat_x/1 -> MATLAB Function/11(x)
  A/1 -> MATLAB Function/14(A)
  B/1 -> MATLAB Function/15(B)
  C/1 -> MATLAB Function/16(C)
  u/1 -> Demux/1
  s/1 -> MATLAB Function/12(s)
  a/1 -> MATLAB Function/13(a)
  Demux/1 -> MATLAB Function/1(u10)
  Demux/2 -> MATLAB Function/2(u9)
  Demux/3 -> MATLAB Function/3(u8)
  Demux/4 -> MATLAB Function/4(u7)
  Demux/5 -> MATLAB Function/5(u6)
  Demux/6 -> MATLAB Function/6(u5)
  Demux/7 -> MATLAB Function/7(u4)
  Demux/8 -> MATLAB Function/8(u3)
  Demux/9 -> MATLAB Function/9(u2)
  Demux/10 -> MATLAB Function/10(u1)

== system MAS_pc_up/Ps2a1 ==
  u : Inport
  hat_x : Inport  Port=2
  A : Constant  Value=A2  VectorParams1D=off
  B : Constant  Value=B2  VectorParams1D=off
  C : Constant  Value=C2  VectorParams1D=off
  Demux : Demux  Outputs=10
  MATLAB Function : MATLAB Function  TreatAsAtomicUnit=on
  a : Constant  Value=a
  s : Constant  Value=s
  hat_x_s : Outport
  hat_y_s : Outport  Port=2
  wires:
  MATLAB Function/2(y) -> hat_y_s/1
  MATLAB Function/1(x_) -> hat_x_s/1
  hat_x/1 -> MATLAB Function/11(x)
  A/1 -> MATLAB Function/14(A)
  B/1 -> MATLAB Function/15(B)
  C/1 -> MATLAB Function/16(C)
  u/1 -> Demux/1
  s/1 -> MATLAB Function/12(s)
  a/1 -> MATLAB Function/13(a)
  Demux/1 -> MATLAB Function/1(u10)
  Demux/2 -> MATLAB Function/2(u9)
  Demux/3 -> MATLAB Function/3(u8)
  Demux/4 -> MATLAB Function/4(u7)
  Demux/5 -> MATLAB Function/5(u6)
  Demux/6 -> MATLAB Function/6(u5)
  Demux/7 -> MATLAB Function/7(u4)
  Demux/8 -> MATLAB Function/8(u3)
  Demux/9 -> MATLAB Function/9(u2)
  Demux/10 -> MATLAB Function/10(u1)

== system MAS_pc_up/Ps2a2 ==
  u : Inport
  hat_x : Inport  Port=2
  A : Constant  Value=A2  VectorParams1D=off
  B : Constant  Value=B2  VectorParams1D=off
  C : Constant  Value=C2  VectorParams1D=off
  Demux : Demux  Outputs=10
  MATLAB Function : MATLAB Function  TreatAsAtomicUnit=on
  a : Constant  Value=a
  s : Constant  Value=s
  hat_x_s : Outport
  hat_y_s : Outport  Port=2
  wires:
  MATLAB Function/2(y) -> hat_y_s/1
  MATLAB Function/1(x_) -> hat_x_s/1
  hat_x/1 -> MATLAB Function/11(x)
  A/1 -> MATLAB Function/14(A)
  B/1 -> MATLAB Function/15(B)
  C/1 -> MATLAB Function/16(C)
  u/1 -> Demux/1
  s/1 -> MATLAB Function/12(s)
  a/1 -> MATLAB Function/13(a)
  Demux/1 -> MATLAB Function/1(u10)
  Demux/2 -> MATLAB Function/2(u9)
  Demux/3 -> MATLAB Function/3(u8)
  Demux/4 -> MATLAB Function/4(u7)
  Demux/5 -> MATLAB Function/5(u6)
  Demux/6 -> MATLAB Function/6(u5)
  Demux/7 -> MATLAB Function/7(u4)
  Demux/8 -> MATLAB Function/8(u3)
  Demux/9 -> MATLAB Function/9(u2)
  Demux/10 -> MATLAB Function/10(u1)

== system MAS_pc_up/Ps2a3 ==
  u : Inport
  hat_x : Inport  Port=2
  A : Constant  Value=A2  VectorParams1D=off
  B : Constant  Value=B2  VectorParams1D=off
  C : Constant  Value=C2  VectorParams1D=off
  Demux : Demux  Outputs=10
  MATLAB Function : MATLAB Function  TreatAsAtomicUnit=on
  a : Constant  Value=a
  s : Constant  Value=s
  hat_x_s : Outport
  hat_y_s : Outport  Port=2
  wires:
  MATLAB Function/2(y) -> hat_y_s/1
  MATLAB Function/1(x_) -> hat_x_s/1
  hat_x/1 -> MATLAB Function/11(x)
  A/1 -> MATLAB Function/14(A)
  B/1 -> MATLAB Function/15(B)
  C/1 -> MATLAB Function/16(C)
  u/1 -> Demux/1
  s/1 -> MATLAB Function/12(s)
  a/1 -> MATLAB Function/13(a)
  Demux/1 -> MATLAB Function/1(u10)
  Demux/2 -> MATLAB Function/2(u9)
  Demux/3 -> MATLAB Function/3(u8)
  Demux/4 -> MATLAB Function/4(u7)
  Demux/5 -> MATLAB Function/5(u6)
  Demux/6 -> MATLAB Function/6(u5)
  Demux/7 -> MATLAB Function/7(u4)
  Demux/8 -> MATLAB Function/8(u3)
  Demux/9 -> MATLAB Function/9(u2)
  Demux/10 -> MATLAB Function/10(u1)

== system MAS_pc_up/Ps3a1 ==
  u : Inport
  hat_x : Inport  Port=2
  A : Constant  Value=A3  VectorParams1D=off
  B : Constant  Value=B3  VectorParams1D=off
  C : Constant  Value=C3  VectorParams1D=off
  Demux : Demux  Outputs=10
  MATLAB Function : MATLAB Function  TreatAsAtomicUnit=on
  a : Constant  Value=a
  s : Constant  Value=s
  hat_x_s : Outport
  hat_y_s : Outport  Port=2
  wires:
  MATLAB Function/2(y) -> hat_y_s/1
  MATLAB Function/1(x_) -> hat_x_s/1
  hat_x/1 -> MATLAB Function/11(x)
  A/1 -> MATLAB Function/14(A)
  B/1 -> MATLAB Function/15(B)
  C/1 -> MATLAB Function/16(C)
  u/1 -> Demux/1
  s/1 -> MATLAB Function/12(s)
  a/1 -> MATLAB Function/13(a)
  Demux/1 -> MATLAB Function/1(u10)
  Demux/2 -> MATLAB Function/2(u9)
  Demux/3 -> MATLAB Function/3(u8)
  Demux/4 -> MATLAB Function/4(u7)
  Demux/5 -> MATLAB Function/5(u6)
  Demux/6 -> MATLAB Function/6(u5)
  Demux/7 -> MATLAB Function/7(u4)
  Demux/8 -> MATLAB Function/8(u3)
  Demux/9 -> MATLAB Function/9(u2)
  Demux/10 -> MATLAB Function/10(u1)

== system MAS_pc_up/Ps3a2 ==
  u : Inport
  hat_x : Inport  Port=2
  A : Constant  Value=A3  VectorParams1D=off
  B : Constant  Value=B3  VectorParams1D=off
  C : Constant  Value=C3  VectorParams1D=off
  Demux : Demux  Outputs=10
  MATLAB Function : MATLAB Function  TreatAsAtomicUnit=on
  a : Constant  Value=a
  s : Constant  Value=s
  hat_x_s : Outport
  hat_y_s : Outport  Port=2
  wires:
  MATLAB Function/2(y) -> hat_y_s/1
  MATLAB Function/1(x_) -> hat_x_s/1
  hat_x/1 -> MATLAB Function/11(x)
  A/1 -> MATLAB Function/14(A)
  B/1 -> MATLAB Function/15(B)
  C/1 -> MATLAB Function/16(C)
  u/1 -> Demux/1
  s/1 -> MATLAB Function/12(s)
  a/1 -> MATLAB Function/13(a)
  Demux/1 -> MATLAB Function/1(u10)
  Demux/2 -> MATLAB Function/2(u9)
  Demux/3 -> MATLAB Function/3(u8)
  Demux/4 -> MATLAB Function/4(u7)
  Demux/5 -> MATLAB Function/5(u6)
  Demux/6 -> MATLAB Function/6(u5)
  Demux/7 -> MATLAB Function/7(u4)
  Demux/8 -> MATLAB Function/8(u3)
  Demux/9 -> MATLAB Function/9(u2)
  Demux/10 -> MATLAB Function/10(u1)

== system MAS_pc_up/Ps3a3 ==
  u : Inport
  hat_x : Inport  Port=2
  A : Constant  Value=A3  VectorParams1D=off
  B : Constant  Value=B3  VectorParams1D=off
  C : Constant  Value=C3  VectorParams1D=off
  Demux : Demux  Outputs=10
  MATLAB Function : MATLAB Function  TreatAsAtomicUnit=on
  a : Constant  Value=a
  s : Constant  Value=s
  hat_x_s : Outport
  hat_y_s : Outport  Port=2
  wires:
  MATLAB Function/2(y) -> hat_y_s/1
  MATLAB Function/1(x_) -> hat_x_s/1
  hat_x/1 -> MATLAB Function/11(x)
  A/1 -> MATLAB Function/14(A)
  B/1 -> MATLAB Function/15(B)
  C/1 -> MATLAB Function/16(C)
  u/1 -> Demux/1
  s/1 -> MATLAB Function/12(s)
  a/1 -> MATLAB Function/13(a)
  Demux/1 -> MATLAB Function/1(u10)
  Demux/2 -> MATLAB Function/2(u9)
  Demux/3 -> MATLAB Function/3(u8)
  Demux/4 -> MATLAB Function/4(u7)
  Demux/5 -> MATLAB Function/5(u6)
  Demux/6 -> MATLAB Function/6(u5)
  Demux/7 -> MATLAB Function/7(u4)
  Demux/8 -> MATLAB Function/8(u3)
  Demux/9 -> MATLAB Function/9(u2)
  Demux/10 -> MATLAB Function/10(u1)

== system MAS_pc_up/Ps4 ==
  u : Inport
  hat_x : Inport  Port=2
  A : Constant  Value=A1  VectorParams1D=off
  B : Constant  Value=B1  VectorParams1D=off
  C : Constant  Value=C1  VectorParams1D=off
  Demux : Demux  Outputs=5
  MATLAB Function : MATLAB Function  TreatAsAtomicUnit=on
  s : Constant  Value=s
  hat_x_s : Outport
  hat_y_s : Outport  Port=2
  wires:
  MATLAB Function/2(y) -> hat_y_s/1
  MATLAB Function/1(x_) -> hat_x_s/1
  hat_x/1 -> MATLAB Function/6(x)
  s/1 -> MATLAB Function/7(tau)
  A/1 -> MATLAB Function/8(A)
  B/1 -> MATLAB Function/9(B)
  C/1 -> MATLAB Function/10(C)
  u/1 -> Demux/1
  Demux/5 -> MATLAB Function/5(u1)
  Demux/4 -> MATLAB Function/4(u2)
  Demux/3 -> MATLAB Function/3(u3)
  Demux/2 -> MATLAB Function/2(u4)
  Demux/1 -> MATLAB Function/1(u5)

== system MAS_pc_up/Ps5 ==
  u : Inport
  hat_x : Inport  Port=2
  A : Constant  Value=A2  VectorParams1D=off
  B : Constant  Value=B2  VectorParams1D=off
  C : Constant  Value=C2  VectorParams1D=off
  Demux : Demux  Outputs=5
  MATLAB Function : MATLAB Function  TreatAsAtomicUnit=on
  s : Constant  Value=s
  hat_x_s : Outport
  hat_y_s : Outport  Port=2
  wires:
  MATLAB Function/2(y) -> hat_y_s/1
  MATLAB Function/1(x_) -> hat_x_s/1
  hat_x/1 -> MATLAB Function/6(x)
  s/1 -> MATLAB Function/7(tau)
  A/1 -> MATLAB Function/8(A)
  B/1 -> MATLAB Function/9(B)
  C/1 -> MATLAB Function/10(C)
  u/1 -> Demux/1
  Demux/5 -> MATLAB Function/5(u1)
  Demux/4 -> MATLAB Function/4(u2)
  Demux/3 -> MATLAB Function/3(u3)
  Demux/2 -> MATLAB Function/2(u4)
  Demux/1 -> MATLAB Function/1(u5)

== system MAS_pc_up/Ps6 ==
  u : Inport
  hat_x : Inport  Port=2
  A : Constant  Value=A3  VectorParams1D=off
  B : Constant  Value=B3  VectorParams1D=off
  C : Constant  Value=C3  VectorParams1D=off
  Demux : Demux  Outputs=5
  MATLAB Function : MATLAB Function  TreatAsAtomicUnit=on
  s : Constant  Value=s
  hat_x_s : Outport
  hat_y_s : Outport  Port=2
  wires:
  MATLAB Function/2(y) -> hat_y_s/1
  MATLAB Function/1(x_) -> hat_x_s/1
  hat_x/1 -> MATLAB Function/6(x)
  s/1 -> MATLAB Function/7(tau)
  A/1 -> MATLAB Function/8(A)
  B/1 -> MATLAB Function/9(B)
  C/1 -> MATLAB Function/10(C)
  u/1 -> Demux/1
  Demux/5 -> MATLAB Function/5(u1)
  Demux/4 -> MATLAB Function/4(u2)
  Demux/3 -> MATLAB Function/3(u3)
  Demux/2 -> MATLAB Function/2(u4)
  Demux/1 -> MATLAB Function/1(u5)

== system MAS_pc_up/Z1 ==
  ref : Inport
  hat_y : Inport  Port=2
  Add : Sum  Inputs=-++
  Unit Delay : UnitDelay  SampleTime=samp_t  HasFrameUpgradeWarning=on
  z : Outport
  wires:
  Unit Delay/1 -> z/1, Add/3
  hat_y/1 -> Add/2
  ref/1 -> Add/1
  Add/1 -> Unit Delay/1

== system MAS_pc_up/Z10 ==
  ref : Inport
  hat_y : Inport  Port=2
  Add : Sum  Inputs=-++
  Unit Delay : UnitDelay  SampleTime=-1  HasFrameUpgradeWarning=on
  z : Outport
  wires:
  Unit Delay/1 -> z/1, Add/3
  hat_y/1 -> Add/2
  ref/1 -> Add/1
  Add/1 -> Unit Delay/1

== system MAS_pc_up/Z11 ==
  ref : Inport
  hat_y : Inport  Port=2
  Add : Sum  Inputs=-++
  Unit Delay : UnitDelay  SampleTime=-1  HasFrameUpgradeWarning=on
  z : Outport
  wires:
  Unit Delay/1 -> z/1, Add/3
  hat_y/1 -> Add/2
  ref/1 -> Add/1
  Add/1 -> Unit Delay/1

== system MAS_pc_up/Z12 ==
  ref : Inport
  hat_y : Inport  Port=2
  Add : Sum  Inputs=-++
  Unit Delay : UnitDelay  SampleTime=-1  HasFrameUpgradeWarning=on
  z : Outport
  wires:
  Unit Delay/1 -> z/1, Add/3
  hat_y/1 -> Add/2
  ref/1 -> Add/1
  Add/1 -> Unit Delay/1

== system MAS_pc_up/Z2 ==
  ref : Inport
  hat_y : Inport  Port=2
  Add : Sum  Inputs=-++
  Unit Delay : UnitDelay  SampleTime=samp_t  HasFrameUpgradeWarning=on
  z : Outport
  wires:
  Unit Delay/1 -> z/1, Add/3
  hat_y/1 -> Add/2
  ref/1 -> Add/1
  Add/1 -> Unit Delay/1

== system MAS_pc_up/Z3 ==
  ref : Inport
  hat_y : Inport  Port=2
  Add : Sum  Inputs=-++
  Unit Delay : UnitDelay  SampleTime=samp_t  HasFrameUpgradeWarning=on
  z : Outport
  wires:
  Unit Delay/1 -> z/1, Add/3
  hat_y/1 -> Add/2
  ref/1 -> Add/1
  Add/1 -> Unit Delay/1

== system MAS_pc_up/Z4 ==
  ref : Inport
  hat_y : Inport  Port=2
  Add : Sum  Inputs=-++
  Unit Delay : UnitDelay  SampleTime=samp_t  HasFrameUpgradeWarning=on
  z : Outport
  wires:
  Unit Delay/1 -> z/1, Add/3
  hat_y/1 -> Add/2
  ref/1 -> Add/1
  Add/1 -> Unit Delay/1

== system MAS_pc_up/Z5 ==
  ref : Inport
  hat_y : Inport  Port=2
  Add : Sum  Inputs=-++
  Unit Delay : UnitDelay  SampleTime=samp_t  HasFrameUpgradeWarning=on
  z : Outport
  wires:
  Unit Delay/1 -> z/1, Add/3
  hat_y/1 -> Add/2
  ref/1 -> Add/1
  Add/1 -> Unit Delay/1

== system MAS_pc_up/Z6 ==
  ref : Inport
  hat_y : Inport  Port=2
  Add : Sum  Inputs=-++
  Unit Delay : UnitDelay  SampleTime=samp_t  HasFrameUpgradeWarning=on
  z : Outport
  wires:
  Unit Delay/1 -> z/1, Add/3
  hat_y/1 -> Add/2
  ref/1 -> Add/1
  Add/1 -> Unit Delay/1

== system MAS_pc_up/Z7 ==
  ref : Inport
  hat_y : Inport  Port=2
  Add : Sum  Inputs=-++
  Unit Delay : UnitDelay  SampleTime=samp_t  HasFrameUpgradeWarning=on
  z : Outport
  wires:
  Unit Delay/1 -> z/1, Add/3
  hat_y/1 -> Add/2
  ref/1 -> Add/1
  Add/1 -> Unit Delay/1

== system MAS_pc_up/Z8 ==
  ref : Inport
  hat_y : Inport  Port=2
  Add : Sum  Inputs=-++
  Unit Delay : UnitDelay  SampleTime=samp_t  HasFrameUpgradeWarning=on
  z : Outport
  wires:
  Unit Delay/1 -> z/1, Add/3
  hat_y/1 -> Add/2
  ref/1 -> Add/1
  Add/1 -> Unit Delay/1

== system MAS_pc_up/Z9 ==
  ref : Inport
  hat_y : Inport  Port=2
  Add : Sum  Inputs=-++
  Unit Delay : UnitDelay  SampleTime=samp_t  HasFrameUpgradeWarning=on
  z : Outport
  wires:
  Unit Delay/1 -> z/1, Add/3
  hat_y/1 -> Add/2
  ref/1 -> Add/1
  Add/1 -> Unit Delay/1

== system MAS_pc_up/u1 ==
  z : Inport
  hat_Y : Inport  Port=2
  Add : Sum
  Constant1 : Constant  Value=M
  Constant2 : Constant  Value=id
  G : Constant  Value=G1  VectorParams1D=off
  H : Constant  Value=H1  VectorParams1D=off
  MATLAB Function : MATLAB Function  TreatAsAtomicUnit=on
  Product : Product  Multiplication=Matrix(*)
  Product1 : Product  Multiplication=Matrix(*)
  u : Outport
  wires:
  z/1 -> Product/2
  G/1 -> Product/1
  Product/1 -> Add/1
  Add/1 -> u/1
  Constant1/1 -> MATLAB Function/1(M)
  hat_Y/1 -> MATLAB Function/2(hat_Y)
  Constant2/1 -> MATLAB Function/3(id)
  MATLAB Function/1(y) -> Product1/2
  H/1 -> Product1/1
  Product1/1 -> Add/2

== system MAS_pc_up/u10 ==
  z : Inport
  hat_Y : Inport  Port=2
  Add : Sum
  Constant1 : Constant  Value=M
  Constant2 : Constant  Value=id
  G : Constant  Value=G1  VectorParams1D=off
  H : Constant  Value=H1  VectorParams1D=off
  MATLAB Function : MATLAB Function  TreatAsAtomicUnit=on
  Product : Product  Multiplication=Matrix(*)
  Product1 : Product  Multiplication=Matrix(*)
  u : Outport
  wires:
  z/1 -> Product/2
  G/1 -> Product/1
  Product/1 -> Add/1
  Add/1 -> u/1
  Constant1/1 -> MATLAB Function/1(M)
  hat_Y/1 -> MATLAB Function/2(hat_Y)
  Constant2/1 -> MATLAB Function/3(id)
  MATLAB Function/1(y) -> Product1/2
  H/1 -> Product1/1
  Product1/1 -> Add/2

== system MAS_pc_up/u11 ==
  z : Inport
  hat_Y : Inport  Port=2
  Add : Sum
  Constant1 : Constant  Value=M
  Constant2 : Constant  Value=id
  G : Constant  Value=G2  VectorParams1D=off
  H : Constant  Value=H2  VectorParams1D=off
  MATLAB Function : MATLAB Function  TreatAsAtomicUnit=on
  Product : Product  Multiplication=Matrix(*)
  Product1 : Product  Multiplication=Matrix(*)
  u : Outport
  wires:
  z/1 -> Product/2
  G/1 -> Product/1
  Product/1 -> Add/1
  Add/1 -> u/1
  Constant1/1 -> MATLAB Function/1(M)
  hat_Y/1 -> MATLAB Function/2(hat_Y)
  Constant2/1 -> MATLAB Function/3(id)
  MATLAB Function/1(y) -> Product1/2
  H/1 -> Product1/1
  Product1/1 -> Add/2

== system MAS_pc_up/u12 ==
  z : Inport
  hat_Y : Inport  Port=2
  Add : Sum
  Constant1 : Constant  Value=M
  Constant2 : Constant  Value=id
  G : Constant  Value=G3  VectorParams1D=off
  H : Constant  Value=H3  VectorParams1D=off
  MATLAB Function : MATLAB Function  TreatAsAtomicUnit=on
  Product : Product  Multiplication=Matrix(*)
  Product1 : Product  Multiplication=Matrix(*)
  u : Outport
  wires:
  z/1 -> Product/2
  G/1 -> Product/1
  Product/1 -> Add/1
  Add/1 -> u/1
  Constant1/1 -> MATLAB Function/1(M)
  hat_Y/1 -> MATLAB Function/2(hat_Y)
  Constant2/1 -> MATLAB Function/3(id)
  MATLAB Function/1(y) -> Product1/2
  H/1 -> Product1/1
  Product1/1 -> Add/2

== system MAS_pc_up/u2 ==
  z : Inport
  hat_Y : Inport  Port=2
  Add : Sum
  Constant1 : Constant  Value=M
  Constant2 : Constant  Value=id
  G : Constant  Value=G2  VectorParams1D=off
  H : Constant  Value=H2  VectorParams1D=off
  MATLAB Function : MATLAB Function  TreatAsAtomicUnit=on
  Product : Product  Multiplication=Matrix(*)
  Product1 : Product  Multiplication=Matrix(*)
  u : Outport
  wires:
  z/1 -> Product/2
  G/1 -> Product/1
  Product/1 -> Add/1
  Add/1 -> u/1
  Constant1/1 -> MATLAB Function/1(M)
  hat_Y/1 -> MATLAB Function/2(hat_Y)
  Constant2/1 -> MATLAB Function/3(id)
  MATLAB Function/1(y) -> Product1/2
  H/1 -> Product1/1
  Product1/1 -> Add/2

== system MAS_pc_up/u3 ==
  z : Inport
  hat_Y : Inport  Port=2
  Add : Sum
  Constant1 : Constant  Value=M
  Constant2 : Constant  Value=id
  G : Constant  Value=G3  VectorParams1D=off
  H : Constant  Value=H3  VectorParams1D=off
  MATLAB Function : MATLAB Function  TreatAsAtomicUnit=on
  Product : Product  Multiplication=Matrix(*)
  Product1 : Product  Multiplication=Matrix(*)
  u : Outport
  wires:
  z/1 -> Product/2
  G/1 -> Product/1
  Product/1 -> Add/1
  Add/1 -> u/1
  Constant1/1 -> MATLAB Function/1(M)
  hat_Y/1 -> MATLAB Function/2(hat_Y)
  Constant2/1 -> MATLAB Function/3(id)
  MATLAB Function/1(y) -> Product1/2
  H/1 -> Product1/1
  Product1/1 -> Add/2

== system MAS_pc_up/u4 ==
  z : Inport
  hat_Y : Inport  Port=2
  Add : Sum
  Constant1 : Constant  Value=M
  Constant2 : Constant  Value=id
  G : Constant  Value=G1  VectorParams1D=off
  H : Constant  Value=H1  VectorParams1D=off
  MATLAB Function : MATLAB Function  TreatAsAtomicUnit=on
  Product : Product  Multiplication=Matrix(*)
  Product1 : Product  Multiplication=Matrix(*)
  u : Outport
  wires:
  z/1 -> Product/2
  G/1 -> Product/1
  Product/1 -> Add/1
  Add/1 -> u/1
  Constant1/1 -> MATLAB Function/1(M)
  hat_Y/1 -> MATLAB Function/2(hat_Y)
  Constant2/1 -> MATLAB Function/3(id)
  MATLAB Function/1(y) -> Product1/2
  H/1 -> Product1/1
  Product1/1 -> Add/2

== system MAS_pc_up/u5 ==
  z : Inport
  hat_Y : Inport  Port=2
  Add : Sum
  Constant1 : Constant  Value=M
  Constant2 : Constant  Value=id
  G : Constant  Value=G2  VectorParams1D=off
  H : Constant  Value=H2  VectorParams1D=off
  MATLAB Function : MATLAB Function  TreatAsAtomicUnit=on
  Product : Product  Multiplication=Matrix(*)
  Product1 : Product  Multiplication=Matrix(*)
  u : Outport
  wires:
  z/1 -> Product/2
  G/1 -> Product/1
  Product/1 -> Add/1
  Add/1 -> u/1
  Constant1/1 -> MATLAB Function/1(M)
  hat_Y/1 -> MATLAB Function/2(hat_Y)
  Constant2/1 -> MATLAB Function/3(id)
  MATLAB Function/1(y) -> Product1/2
  H/1 -> Product1/1
  Product1/1 -> Add/2

== system MAS_pc_up/u6 ==
  z : Inport
  hat_Y : Inport  Port=2
  Add : Sum
  Constant1 : Constant  Value=M
  Constant2 : Constant  Value=id
  G : Constant  Value=G3  VectorParams1D=off
  H : Constant  Value=H3  VectorParams1D=off
  MATLAB Function : MATLAB Function  TreatAsAtomicUnit=on
  Product : Product  Multiplication=Matrix(*)
  Product1 : Product  Multiplication=Matrix(*)
  u : Outport
  wires:
  z/1 -> Product/2
  G/1 -> Product/1
  Product/1 -> Add/1
  Add/1 -> u/1
  Constant1/1 -> MATLAB Function/1(M)
  hat_Y/1 -> MATLAB Function/2(hat_Y)
  Constant2/1 -> MATLAB Function/3(id)
  MATLAB Function/1(y) -> Product1/2
  H/1 -> Product1/1
  Product1/1 -> Add/2
